simulink model "amplificator"  (R2017b)
settings: Solver=VariableStepAuto  StartTime=0.0  StopTime=10.0  RelTol=1e-3
settings Model: Creator=alinvoicu26  LastModifiedBy=alinvoicu26

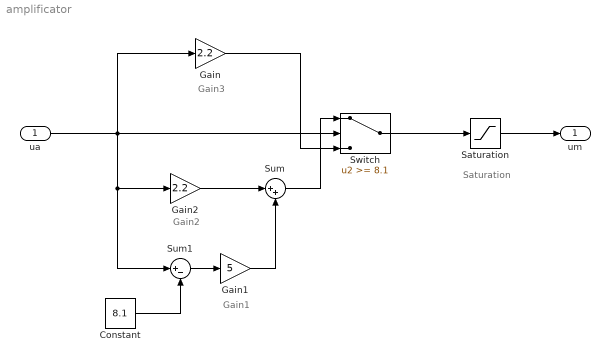
== system amplificator ==
  note: Saturation
  note: Gain3
  note: Gain2
  note: Gain1
  "ua " : Inport
  Constant : Constant  Value=8.1
  Gain : Gain  Gain=2.2
  Gain1 : Gain  Gain=5
  Gain2 : Gain  Gain=2.2
  Saturation : Saturate  UpperLimit=22  LowerLimit=0
  Sum : Sum  Inputs=|++
  Sum1 : Sum  Inputs=|+-
  Switch : Switch  Threshold=8.1
  "um " : Outport
  wires:
  "ua "/1 -> Sum1/1, Gain2/1, Gain/1, Switch/2
  Switch/1 -> Saturation/1
  Gain2/1 -> Sum/1
  Sum/1 -> Switch/1
  Gain/1 -> Switch/3
  Gain1/1 -> Sum/2
  Sum1/1 -> Gain1/1
  Constant/1 -> Sum1/2
  Saturation/1 -> "um "/1
